simulink model "control_nolineal_entrada_estado_2"  (R2018a)
settings: Solver=VariableStepAuto  StartTime=0.0  StopTime=10.0  RelTol=1e-3
InitFcn:
  | control_nolineal_linealizacion_entrada_estado2
values from neighbouring files (symbols this model uses):
  kii = kt(1,3)    [control_nolineal_linealizacion_entrada_estado.m]    (also in control_nolineal_linealizacion_entrada_estado2.m)
  kpi = kt(1,1:2)    [control_nolineal_linealizacion_entrada_estado.m]    (also in control_nolineal_linealizacion_entrada_estado2.m)
libraries: simulink x1
settings Model: Creator=carma  LastModifiedBy=carma

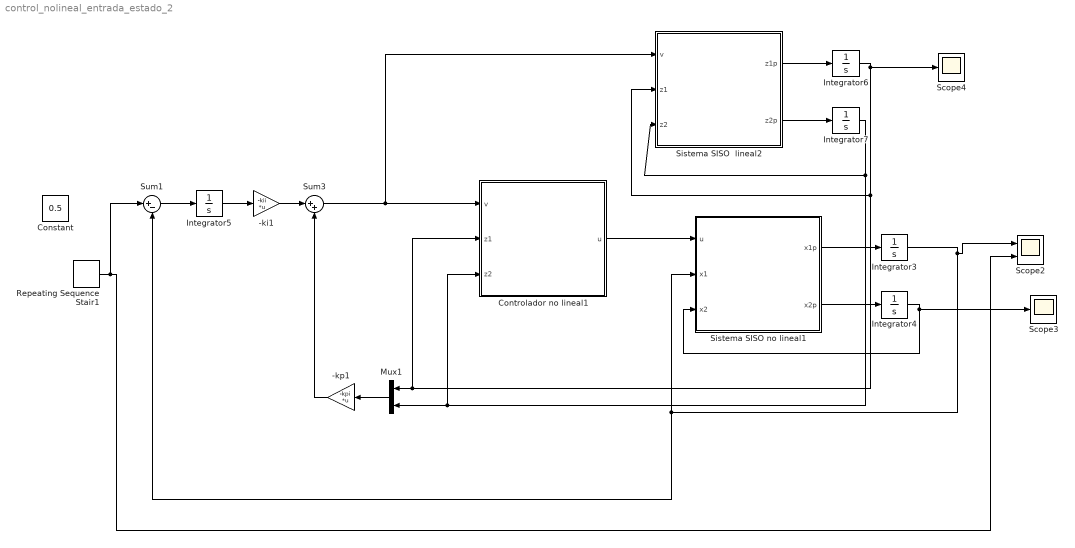
== system control_nolineal_entrada_estado_2 ==
  -ki1 : Gain  Gain=-kii  Multiplication=Matrix(K*u) (u vector)
  -kp1 : Gain  Gain=-kpi  Multiplication=Matrix(K*u) (u vector)
  Constant : Constant  Value=0.5
  Controlador no lineal1 : MATLAB Function  TreatAsAtomicUnit=on
  Integrator{3..7} (5 alike) : Integrator
  Mux1 : Mux  Inputs=2
  Repeating Sequence Stair1 : simulink/Sources/Repeating Sequence Stair  OutValues=[0.5 0.4 0.2 0.3 0.4].'  tsamp=0.75  OutMin=[]  OutMax=[]  OutDataTypeStr=double  OutputDataTypeScalingMode=double  OutDataType=fixdt(0,8)  ConRadixGroup=Best Precision: Vector-wise  OutScaling=2^-12
  Scope2 : Scope  NumInputPorts=2
  Scope3 : Scope
  Scope4 : Scope
  Sistema SISO  lineal2 : MATLAB Function  TreatAsAtomicUnit=on
  Sistema SISO no lineal1 : MATLAB Function  TreatAsAtomicUnit=on
  Sum1 : Sum  Inputs=|+-
  Sum3 : Sum  Inputs=|++
  wires:
  Repeating Sequence Stair1/1 -> Sum1/1, Scope2/2
  Sum3/1 -> Sistema SISO  lineal2/1(v), Controlador no lineal1/1(v)
  -kp1/1 -> Sum3/2
  Sum1/1 -> Integrator5/1
  Integrator3/1 -> Scope2/1, Sum1/2, Sistema SISO no lineal1/2(x1)
  Integrator4/1 -> Scope3/1, Sistema SISO no lineal1/3(x2)
  Integrator5/1 -> -ki1/1
  Sistema SISO no lineal1/1(x1p) -> Integrator3/1
  -ki1/1 -> Sum3/1
  Mux1/1 -> -kp1/1
  Sistema SISO no lineal1/2(x2p) -> Integrator4/1
  Controlador no lineal1/1(u) -> Sistema SISO no lineal1/1(u)
  Sistema SISO  lineal2/1(z1p) -> Integrator6/1
  Sistema SISO  lineal2/2(z2p) -> Integrator7/1
  Integrator6/1 -> Scope4/1, Sistema SISO  lineal2/2(z1), Controlador no lineal1/2(z1), Mux1/1
  Integrator7/1 -> Sistema SISO  lineal2/3(z2), Controlador no lineal1/3(z2), Mux1/2

== matlab function control_nolineal_entrada_estado_2/Controlador no lineal1 ==
  data: v input; u output; z1 input; z2 input
function u = fcn(v,z1,z2)

%parametros
a=4;


u=(v+2*z1*cos(z1)-cos(z1)*sin(z1))/(a*cos(2*z1));

%s=5;
%syms y
%Cx3=(2+10^(pk2-y))/(1+10^(pk2-y)+10^(pk1+pk2-2*y));
%h=-x1+x2-x3*Cx3+10^(-y)-10^(y-pkw)==0;

%s=double(solve(h));

== matlab function control_nolineal_entrada_estado_2/Sistema SISO no lineal1 ==
  data: u input; x1p output; x1 input; x2 input; x2p output
function [x1p,x2p]= fcn(u,x1,x2)


a=4;


x1p=-2*x1+a*x2+sin(x1);
x2p=-x2*cos(x1)+u*cos(2*x1);
%s=5;
%syms y
%Cx3=(2+10^(pk2-y))/(1+10^(pk2-y)+10^(pk1+pk2-2*y));
%h=-x1+x2-x3*Cx3+10^(-y)-10^(y-pkw)==0;

%s=double(solve(h));

== matlab function control_nolineal_entrada_estado_2/Sistema SISO  lineal2 ==
  data: v input; z1p output; z1 input; z2 input; z2p output
function [z1p,z2p]= fcn(v,z1,z2)

%parametros
a=4;



z1p=-2*z1+z2;
z2p=v;

%s=5;
%syms y
%Cx3=(2+10^(pk2-y))/(1+10^(pk2-y)+10^(pk1+pk2-2*y));
%h=-x1+x2-x3*Cx3+10^(-y)-10^(y-pkw)==0;

%s=double(solve(h));
